simulink model "god"  (R2018a)
settings: Solver=VariableStepAuto  StartTime=0.0  StopTime=10  FixedStep=0.01  RelTol=1e-3
libraries: instrumentlib x15
settings Model: EnablePacing=on  Creator=U500304  LastModifiedBy=U500304
settings SolverCC: ZeroCrossAlgorithm=Adaptive
settings DataIOCC: SaveOutput=off  SaveTime=off
settings DebuggingCC: MaxConsecutiveZCsMsg=none

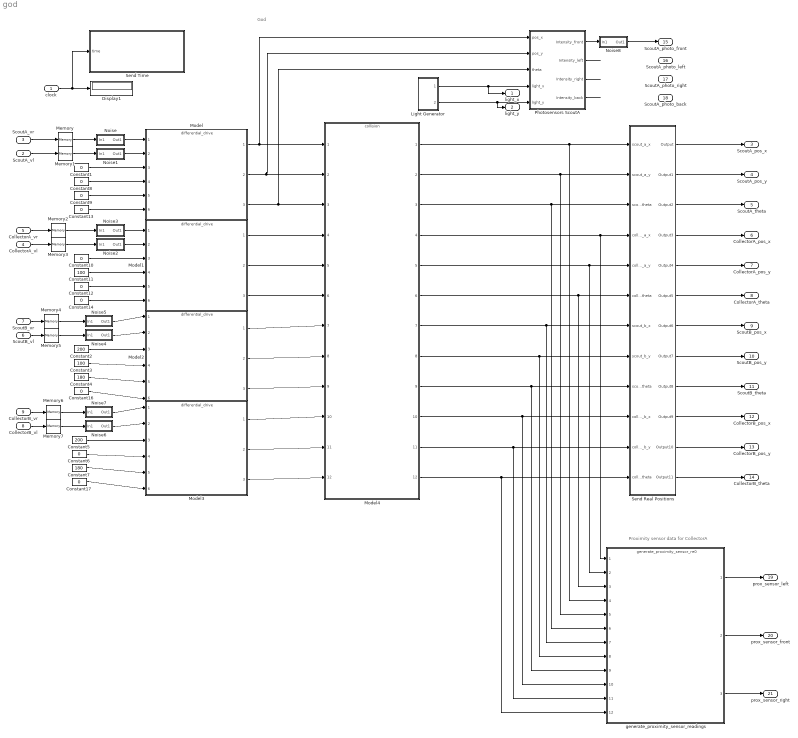
== system god ==
  note: Proximity sensor data for CollectorA
  note: God
  clock : Inport  OutDataTypeStr=double  PortDimensions=1  SampleTime=0
  ScoutA_vl : Inport  Port=2
  ScoutA_vr : Inport  Port=3
  CollectorA_vl : Inport  Port=4
  CollectorA_vr : Inport  Port=5
  ScoutB_vl : Inport  Port=6
  ScoutB_vr : Inport  Port=7
  CollectorB_vl : Inport  Port=8
  CollectorB_vr : Inport  Port=9
  Constant{1,6,8..10,12..14,16..17} (10 alike) : Constant  Value=0
  Constant11 : Constant  Value=100
  Constant2 : Constant  Value=200
  Constant3 : Constant  Value=100
  Constant4 : Constant  Value=180
  Constant5 : Constant  Value=200
  Constant7 : Constant  Value=180
  Display1 : Display
  Light Generator : Subsystem
  Memory{,1..7} (8 alike) : Memory
  Model{,1..3} (4 alike) : ModelReference  ModelNameDialog=differential_drive.slx  SimulationMode=Normal  ModelReferenceVersion=1.313
  Model4 : ModelReference  ModelNameDialog=collision.slx  SimulationMode=Normal  ModelReferenceVersion=1.672
  Noise : Subsystem
  Noise1 : Subsystem
  Noise2 : Subsystem
  Noise3 : Subsystem
  Noise4 : Subsystem
  Noise5 : Subsystem
  Noise6 : Subsystem
  Noise7 : Subsystem
  Noise8 : Subsystem
  Photosensors ScoutA : Subsystem
  Send Real Positions : Subsystem
  Send Time : Subsystem
  generate_proximity_sensor_readings : ModelReference  ModelNameDialog=generate_proximity_sensor_re0  SimulationMode=Normal  ModelReferenceVersion=1.659
  light_x : Outport
  light_y : Outport  Port=2
  ScoutA_pos_x : Outport  Port=3
  ScoutA_pos_y : Outport  Port=4
  ScoutA_theta : Outport  Port=5
  CollectorA_pos_x : Outport  Port=6
  CollectorA_pos_y : Outport  Port=7
  CollectorA_theta : Outport  Port=8
  ScoutB_pos_x : Outport  Port=9
  ScoutB_pos_y : Outport  Port=10
  ScoutB_theta : Outport  Port=11
  CollectorB_pos_x : Outport  Port=12
  CollectorB_pos_y : Outport  Port=13
  CollectorB_theta : Outport  Port=14
  ScoutA_photo_front : Outport  Port=15
  ScoutA_photo_left : Outport  Port=16
  ScoutA_photo_right : Outport  Port=17
  ScoutA_photo_back : Outport  Port=18
  prox_sensor_left : Outport  Port=19
  prox_sensor_front : Outport  Port=20
  prox_sensor_right : Outport  Port=21
  wires:
  clock/1 -> Send Time/1(time), Display1/1
  Constant9/1 -> Model/5
  Constant1/1 -> Model/3
  Constant8/1 -> Model/4
  Constant11/1 -> Model1/4
  Constant10/1 -> Model1/3
  Constant12/1 -> Model1/5
  ScoutB_vl/1 -> Memory5/1
  ScoutB_vr/1 -> Memory4/1
  Constant4/1 -> Model2/5
  Constant2/1 -> Model2/3
  Constant3/1 -> Model2/4
  Constant6/1 -> Model3/4
  Constant7/1 -> Model3/5
  Constant5/1 -> Model3/3
  CollectorB_vl/1 -> Memory7/1
  CollectorB_vr/1 -> Memory6/1
  Noise5/1(Out1) -> Model2/1
  Noise4/1(Out1) -> Model2/2
  Noise6/1(Out1) -> Model3/2
  Noise7/1(Out1) -> Model3/1
  Light Generator/1(Light_x) -> light_x/1, Photosensors ScoutA/4(light_x)
  Light Generator/2(Light_y) -> light_y/1, Photosensors ScoutA/5(light_y)
  Photosensors ScoutA/1(Intensity_front) -> Noise8/1(In1)
  Photosensors ScoutA/2(Intensity_left) -> ?
  Photosensors ScoutA/3(Intensity_right) -> ?
  Photosensors ScoutA/4(Intensity_back) -> ?
  Noise/1(Out1) -> Model/1
  Noise1/1(Out1) -> Model/2
  Noise2/1(Out1) -> Model1/2
  Noise3/1(Out1) -> Model1/1
  Model/3 -> Photosensors ScoutA/3(theta), Model4/3
  Model/2 -> Photosensors ScoutA/2(pos_y), Model4/2
  Model/1 -> Photosensors ScoutA/1(pos_x), Model4/1
  ScoutA_vr/1 -> Memory/1
  ScoutA_vl/1 -> Memory1/1
  CollectorA_vr/1 -> Memory2/1
  CollectorA_vl/1 -> Memory3/1
  Memory/1 -> Noise/1(In1)
  Memory1/1 -> Noise1/1(In1)
  Memory2/1 -> Noise3/1(In1)
  Memory3/1 -> Noise2/1(In1)
  Constant13/1 -> Model/6
  Constant14/1 -> Model1/6
  Constant16/1 -> Model2/6
  Constant17/1 -> Model3/6
  Model4/11 -> generate_proximity_sensor_readings/11, Send Real Positions/11(collector_b_y)
  Model4/10 -> generate_proximity_sensor_readings/10, Send Real Positions/10(collector_b_x)
  Model4/9 -> generate_proximity_sensor_readings/9, Send Real Positions/9(scout_b_theta)
  Model4/8 -> generate_proximity_sensor_readings/8, Send Real Positions/8(scout_b_y)
  Model4/7 -> generate_proximity_sensor_readings/7, Send Real Positions/7(scout_b_x)
  Model4/12 -> generate_proximity_sensor_readings/12, Send Real Positions/12(collector_b_theta)
  Memory5/1 -> Noise4/1(In1)
  Memory4/1 -> Noise5/1(In1)
  Memory6/1 -> Noise7/1(In1)
  Memory7/1 -> Noise6/1(In1)
  Model1/1 -> Model4/4
  Model1/2 -> Model4/5
  Model1/3 -> Model4/6
  Model2/1 -> Model4/7
  Model2/2 -> Model4/8
  Model2/3 -> Model4/9
  Model3/1 -> Model4/10
  Model3/2 -> Model4/11
  Model3/3 -> Model4/12
  Send Real Positions/1(Output) -> ScoutA_pos_x/1
  Send Real Positions/2(Output1) -> ScoutA_pos_y/1
  Send Real Positions/3(Output2) -> ScoutA_theta/1
  Send Real Positions/4(Output3) -> CollectorA_pos_x/1
  Send Real Positions/5(Output4) -> CollectorA_pos_y/1
  Send Real Positions/6(Output5) -> CollectorA_theta/1
  Send Real Positions/7(Output6) -> ScoutB_pos_x/1
  Send Real Positions/8(Output7) -> ScoutB_pos_y/1
  Send Real Positions/9(Output8) -> ScoutB_theta/1
  Send Real Positions/10(Output9) -> CollectorB_pos_x/1
  Send Real Positions/11(Output10) -> CollectorB_pos_y/1
  Send Real Positions/12(Output11) -> CollectorB_theta/1
  Model4/2 -> generate_proximity_sensor_readings/5, Send Real Positions/2(scout_a_y)
  Model4/3 -> generate_proximity_sensor_readings/6, Send Real Positions/3(scout_a_theta)
  Model4/4 -> generate_proximity_sensor_readings/1, Send Real Positions/4(collector_a_x)
  Model4/5 -> generate_proximity_sensor_readings/2, Send Real Positions/5(collector_a_y)
  Model4/6 -> generate_proximity_sensor_readings/3, Send Real Positions/6(collector_a_theta)
  generate_proximity_sensor_readings/1 -> prox_sensor_left/1
  generate_proximity_sensor_readings/2 -> prox_sensor_front/1
  generate_proximity_sensor_readings/3 -> prox_sensor_right/1
  Model4/1 -> generate_proximity_sensor_readings/4, Send Real Positions/1(scout_a_x)
  Noise8/1(Out1) -> ScoutA_photo_front/1
  ? -> ScoutA_photo_left/1
  ? -> ScoutA_photo_right/1
  ? -> ScoutA_photo_back/1

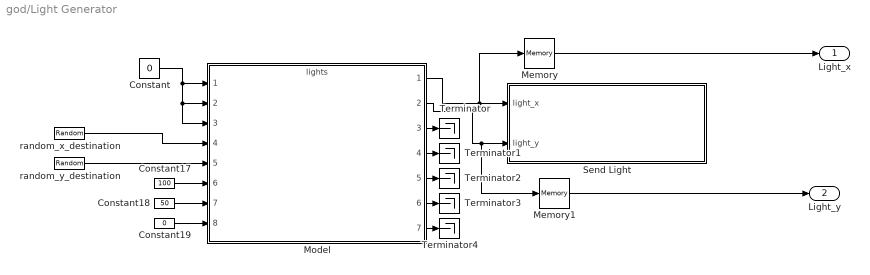
== system god/Light Generator ==
  Constant : Constant  Value=0
  Constant17 : Constant  Value=100
  Constant18 : Constant  Value=50
  Constant19 : Constant  Value=0
  Memory : Memory
  Memory1 : Memory
  Model : ModelReference  ModelNameDialog=lights  SimulationMode=Normal  ModelReferenceVersion=1.293
  Send Light : Subsystem
  Terminator{,1..4} (5 alike) : Terminator
  random_x_destination : UniformRandomNumber  Minimum=0  Maximum=199  Seed=14  SampleTime=1
  random_y_destination : UniformRandomNumber  Minimum=0  Maximum=99  Seed=66  SampleTime=1
  Light_x : Outport
  Light_y : Outport  Port=2
  wires:
  Model/3 -> Terminator/1
  Constant17/1 -> Model/6
  random_y_destination/1 -> Model/5
  Model/6 -> Terminator3/1
  Constant19/1 -> Model/8
  Memory1/1 -> Light_y/1
  Constant/1 -> Model/1, Model/3, Model/2
  Model/4 -> Terminator1/1
  Model/1 -> Memory/1, Send Light/1(light_x)
  Model/2 -> Memory1/1, Send Light/2(light_y)
  random_x_destination/1 -> Model/4
  Model/5 -> Terminator2/1
  Model/7 -> Terminator4/1
  Constant18/1 -> Model/7
  Memory/1 -> Light_x/1

== system god/Noise ==
  In1 : Inport
  Add : Sum
  Multiply : Product
  Uniform Random Number : UniformRandomNumber  Minimum=-0.02  Maximum=0.02  SampleTime=0.1
  Out1 : Outport
  wires:
  Multiply/1 -> Add/1
  In1/1 -> Add/2, Multiply/2
  Uniform Random Number/1 -> Multiply/1
  Add/1 -> Out1/1

== system god/Noise1 ==
  In1 : Inport
  Add : Sum
  Multiply : Product
  Uniform Random Number : UniformRandomNumber  Minimum=-0.02  Maximum=0.02  Seed=1  SampleTime=0.1
  Out1 : Outport
  wires:
  Add/1 -> Out1/1
  Uniform Random Number/1 -> Multiply/1
  In1/1 -> Multiply/2, Add/2
  Multiply/1 -> Add/1

== system god/Noise2 ==
  In1 : Inport
  Add : Sum
  Multiply : Product
  Uniform Random Number : UniformRandomNumber  Minimum=-0.02  Maximum=0.02  SampleTime=0.1
  Out1 : Outport
  wires:
  Add/1 -> Out1/1
  Uniform Random Number/1 -> Multiply/1
  In1/1 -> Multiply/2, Add/2
  Multiply/1 -> Add/1

== system god/Noise3 ==
  In1 : Inport
  Add : Sum
  Multiply : Product
  Uniform Random Number : UniformRandomNumber  Minimum=-0.02  Maximum=0.02  SampleTime=0.1
  Out1 : Outport
  wires:
  Multiply/1 -> Add/1
  In1/1 -> Add/2, Multiply/2
  Uniform Random Number/1 -> Multiply/1
  Add/1 -> Out1/1

== system god/Noise4 ==
  In1 : Inport
  Add : Sum
  Multiply : Product
  Uniform Random Number : UniformRandomNumber  Minimum=-0.02  Maximum=0.02  Seed=2  SampleTime=0.1
  Out1 : Outport
  wires:
  Multiply/1 -> Add/1
  In1/1 -> Add/2, Multiply/2
  Uniform Random Number/1 -> Multiply/1
  Add/1 -> Out1/1

== system god/Noise5 ==
  In1 : Inport
  Add : Sum
  Multiply : Product
  Uniform Random Number : UniformRandomNumber  Minimum=-0.02  Maximum=0.02  Seed=3  SampleTime=0.1
  Out1 : Outport
  wires:
  Add/1 -> Out1/1
  Uniform Random Number/1 -> Multiply/1
  In1/1 -> Multiply/2, Add/2
  Multiply/1 -> Add/1

== system god/Noise6 ==
  In1 : Inport
  Add : Sum
  Multiply : Product
  Uniform Random Number : UniformRandomNumber  Minimum=-0.02  Maximum=0.02  Seed=4  SampleTime=0.1
  Out1 : Outport
  wires:
  Add/1 -> Out1/1
  Uniform Random Number/1 -> Multiply/1
  In1/1 -> Multiply/2, Add/2
  Multiply/1 -> Add/1

== system god/Noise7 ==
  In1 : Inport
  Add : Sum
  Multiply : Product
  Uniform Random Number : UniformRandomNumber  Minimum=-0.02  Maximum=0.02  Seed=5  SampleTime=0.1
  Out1 : Outport
  wires:
  Multiply/1 -> Add/1
  In1/1 -> Add/2, Multiply/2
  Uniform Random Number/1 -> Multiply/1
  Add/1 -> Out1/1

== system god/Noise8 ==
  In1 : Inport
  Add : Sum
  Constant : Constant  Value=255
  Constant1 : Constant  Value=0
  Multiply : Product
  Switch : Switch  Criteria=u2 > Threshold  Threshold=255
  Switch1 : Switch  Criteria=u2 > Threshold
  Uniform Random Number : UniformRandomNumber  Minimum=-0.04  Maximum=0.04  SampleTime=0.1
  Out1 : Outport
  wires:
  Uniform Random Number/1 -> Multiply/1
  In1/1 -> Multiply/2, Add/2
  Multiply/1 -> Add/1
  Add/1 -> Switch/3
  Constant/1 -> Switch/1, Switch/2
  Switch/1 -> Switch1/1
  Constant1/1 -> Switch1/2, Switch1/3
  Switch1/1 -> Out1/1

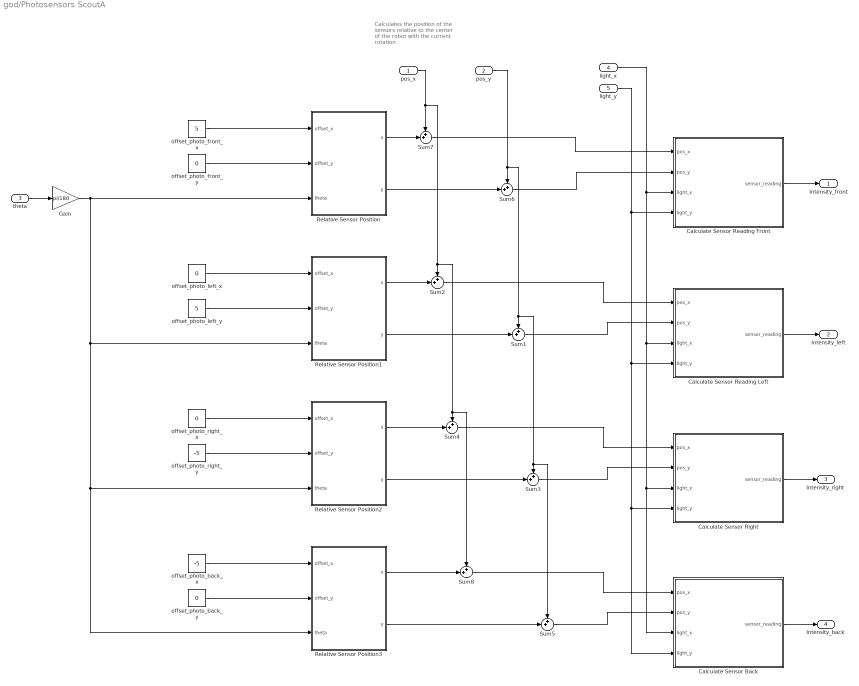
== system god/Photosensors ScoutA ==
  note: Calculates the position of
      | the sensors relative to the
      | center of the robot with the
      | current rotation
  pos_x : Inport
  pos_y : Inport  Port=2
  theta : Inport  Port=3
  light_x : Inport  Port=4
  light_y : Inport  Port=5
  Calculate Sensor Back : Subsystem
  Calculate Sensor Reading Front : Subsystem
  Calculate Sensor Reading Left : Subsystem
  Calculate Sensor Right : Subsystem
  Gain : Gain  Gain=pi/180
  Relative Sensor Position : Subsystem  TreatAsAtomicUnit=on
  Relative Sensor Position1 : Subsystem
  Relative Sensor Position2 : Subsystem
  Relative Sensor Position3 : Subsystem
  Sum{1..8} (8 alike) : Sum  Inputs=++|
  offset_photo_back_x : Constant  Value=-5
  offset_photo_back_y : Constant  Value=0
  offset_photo_front_x : Constant  Value=5
  offset_photo_front_y : Constant  Value=0
  offset_photo_left_x : Constant  Value=0
  offset_photo_left_y : Constant  Value=5
  offset_photo_right_x : Constant  Value=0
  offset_photo_right_y : Constant  Value=-5
  Intensity_front : Outport
  Intensity_left : Outport  Port=2
  Intensity_right : Outport  Port=3
  Intensity_back : Outport  Port=4
  wires:
  offset_photo_front_x/1 -> Relative Sensor Position/1(offset_x)
  offset_photo_front_y/1 -> Relative Sensor Position/2(offset_y)
  Relative Sensor Position/2(y) -> Sum6/2
  Calculate Sensor Reading Front/1(sensor_reading) -> Intensity_front/1
  Sum6/1 -> Calculate Sensor Reading Front/2(pos_y)
  Sum7/1 -> Calculate Sensor Reading Front/1(pos_x)
  offset_photo_left_y/1 -> Relative Sensor Position1/2(offset_y)
  offset_photo_left_x/1 -> Relative Sensor Position1/1(offset_x)
  Relative Sensor Position/1(x) -> Sum7/2
  Relative Sensor Position1/1(x) -> Sum2/2
  Relative Sensor Position1/2(y) -> Sum1/2
  Sum1/1 -> Calculate Sensor Reading Left/2(pos_y)
  Sum2/1 -> Calculate Sensor Reading Left/1(pos_x)
  offset_photo_right_y/1 -> Relative Sensor Position2/2(offset_y)
  offset_photo_right_x/1 -> Relative Sensor Position2/1(offset_x)
  Relative Sensor Position2/1(x) -> Sum4/2
  Sum4/1 -> Calculate Sensor Right/1(pos_x)
  Sum3/1 -> Calculate Sensor Right/2(pos_y)
  Relative Sensor Position2/2(y) -> Sum3/2
  light_y/1 -> Calculate Sensor Back/4(light_y), Calculate Sensor Right/4(light_y), Calculate Sensor Reading Left/4(light_y), Calculate Sensor Reading Front/4(light_y)
  Relative Sensor Position3/2(y) -> Sum5/2
  pos_y/1 -> Sum6/1, Sum5/1, Sum3/1, Sum1/1
  Sum5/1 -> Calculate Sensor Back/2(pos_y)
  Sum8/1 -> Calculate Sensor Back/1(pos_x)
  Gain/1 -> Relative Sensor Position3/3(theta), Relative Sensor Position2/3(theta), Relative Sensor Position1/3(theta), Relative Sensor Position/3(theta)
  Relative Sensor Position3/1(x) -> Sum8/2
  offset_photo_back_x/1 -> Relative Sensor Position3/1(offset_x)
  offset_photo_back_y/1 -> Relative Sensor Position3/2(offset_y)
  light_x/1 -> Calculate Sensor Back/3(light_x), Calculate Sensor Right/3(light_x), Calculate Sensor Reading Left/3(light_x), Calculate Sensor Reading Front/3(light_x)
  pos_x/1 -> Sum8/1, Sum4/1, Sum2/1, Sum7/1
  Calculate Sensor Reading Left/1(sensor_reading) -> Intensity_left/1
  Calculate Sensor Right/1(sensor_reading) -> Intensity_right/1
  Calculate Sensor Back/1(sensor_reading) -> Intensity_back/1
  theta/1 -> Gain/1

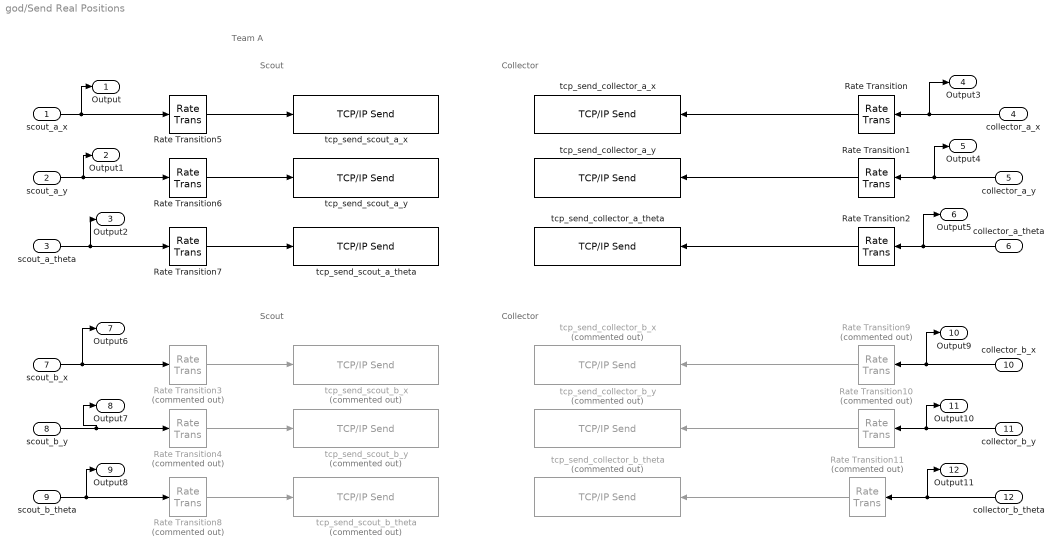
== system god/Send Real Positions ==
  note: Team A
  note: Scout
  note: Collector
  note: Scout
  note: Collector
  scout_a_x : Inport
  scout_a_y : Inport  Port=2
  scout_a_theta : Inport  Port=3
  collector_a_x : Inport  Port=4
  collector_a_y : Inport  Port=5
  collector_a_theta : Inport  Port=6
  scout_b_x : Inport  Port=7
  scout_b_y : Inport  Port=8
  scout_b_theta : Inport  Port=9
  collector_b_x : Inport  Port=10
  collector_b_y : Inport  Port=11
  collector_b_theta : Inport  Port=12
  Rate Transition{,1..2,5..7} (6 alike) : RateTransition  OutPortSampleTime=0.05
  Rate Transition{3..4,8..11} (6 alike) : RateTransition  Commented=on  OutPortSampleTime=0.1
  tcp_send_collector_a_theta : instrumentlib/TCP//IP Send  Host=localhost  Port=50034  EnableBlockingMode=off  Timeout=1  ByteOrder=LittleEndian  TransferDelay=on
      settings: SourceProductName=Instrument Control Toolbox
  tcp_send_collector_a_x : instrumentlib/TCP//IP Send  Host=localhost  Port=50032  EnableBlockingMode=off  Timeout=1  ByteOrder=LittleEndian  TransferDelay=on
      settings: SourceProductName=Instrument Control Toolbox
  tcp_send_collector_a_y : instrumentlib/TCP//IP Send  Host=localhost  Port=50033  EnableBlockingMode=off  Timeout=1  ByteOrder=LittleEndian  TransferDelay=on
      settings: SourceProductName=Instrument Control Toolbox
  tcp_send_collector_b_theta : instrumentlib/TCP//IP Send  Commented=on  Host=localhost  Port=50012  EnableBlockingMode=on  Timeout=1  ByteOrder=LittleEndian  TransferDelay=on
      settings: SourceProductName=Instrument Control Toolbox
  tcp_send_collector_b_x : instrumentlib/TCP//IP Send  Commented=on  Host=localhost  Port=50010  EnableBlockingMode=on  Timeout=1  ByteOrder=LittleEndian  TransferDelay=on
      settings: SourceProductName=Instrument Control Toolbox
  tcp_send_collector_b_y : instrumentlib/TCP//IP Send  Commented=on  Host=localhost  Port=50011  EnableBlockingMode=on  Timeout=1  ByteOrder=LittleEndian  TransferDelay=on
      settings: SourceProductName=Instrument Control Toolbox
  tcp_send_scout_a_theta : instrumentlib/TCP//IP Send  Host=localhost  Port=50031  EnableBlockingMode=off  Timeout=1  ByteOrder=LittleEndian  TransferDelay=on
      settings: SourceProductName=Instrument Control Toolbox
  tcp_send_scout_a_x : instrumentlib/TCP//IP Send  Host=localhost  Port=50029  EnableBlockingMode=off  Timeout=1  ByteOrder=LittleEndian  TransferDelay=on
      settings: SourceProductName=Instrument Control Toolbox
  tcp_send_scout_a_y : instrumentlib/TCP//IP Send  Host=localhost  Port=50030  EnableBlockingMode=off  Timeout=1  ByteOrder=LittleEndian  TransferDelay=on
      settings: SourceProductName=Instrument Control Toolbox
  tcp_send_scout_b_theta : instrumentlib/TCP//IP Send  Commented=on  Host=localhost  Port=50009  EnableBlockingMode=on  Timeout=1  ByteOrder=LittleEndian  TransferDelay=on
      settings: SourceProductName=Instrument Control Toolbox
  tcp_send_scout_b_x : instrumentlib/TCP//IP Send  Commented=on  Host=localhost  Port=50007  EnableBlockingMode=on  Timeout=1  ByteOrder=LittleEndian  TransferDelay=on
      settings: SourceProductName=Instrument Control Toolbox
  tcp_send_scout_b_y : instrumentlib/TCP//IP Send  Commented=on  Host=localhost  Port=50008  EnableBlockingMode=on  Timeout=1  ByteOrder=LittleEndian  TransferDelay=on
      settings: SourceProductName=Instrument Control Toolbox
  Output : Outport
  Output1 : Outport  Port=2
  Output2 : Outport  Port=3
  Output3 : Outport  Port=4
  Output4 : Outport  Port=5
  Output5 : Outport  Port=6
  Output6 : Outport  Port=7
  Output7 : Outport  Port=8
  Output8 : Outport  Port=9
  Output9 : Outport  Port=10
  Output10 : Outport  Port=11
  Output11 : Outport  Port=12
  wires:
  collector_b_x/1 -> Output9/1, Rate Transition9/1
  scout_a_x/1 -> Output/1, Rate Transition5/1
  collector_b_y/1 -> Output10/1, Rate Transition10/1
  scout_a_y/1 -> Output1/1, Rate Transition6/1
  collector_a_y/1 -> Output4/1, Rate Transition1/1
  collector_a_theta/1 -> Output5/1, Rate Transition2/1
  collector_b_theta/1 -> Output11/1, Rate Transition11/1
  scout_a_theta/1 -> Output2/1, Rate Transition7/1
  scout_b_theta/1 -> Output8/1, Rate Transition8/1
  scout_b_y/1 -> Output7/1, Rate Transition4/1
  scout_b_x/1 -> Output6/1, Rate Transition3/1
  Rate Transition/1 -> tcp_send_collector_a_x/1
  Rate Transition1/1 -> tcp_send_collector_a_y/1
  Rate Transition2/1 -> tcp_send_collector_a_theta/1
  Rate Transition5/1 -> tcp_send_scout_a_x/1
  Rate Transition6/1 -> tcp_send_scout_a_y/1
  Rate Transition7/1 -> tcp_send_scout_a_theta/1
  Rate Transition3/1 -> tcp_send_scout_b_x/1
  Rate Transition4/1 -> tcp_send_scout_b_y/1
  Rate Transition8/1 -> tcp_send_scout_b_theta/1
  Rate Transition9/1 -> tcp_send_collector_b_x/1
  Rate Transition10/1 -> tcp_send_collector_b_y/1
  Rate Transition11/1 -> tcp_send_collector_b_theta/1
  collector_a_x/1 -> Output3/1, Rate Transition/1

== system god/Send Time ==
  note: Light
  time : Inport
  Rate Transition8 : RateTransition  OutPortSampleTime=0.1
  tcp_send_light_x : instrumentlib/TCP//IP Send  Host=localhost  Port=50021  EnableBlockingMode=on  Timeout=1  ByteOrder=LittleEndian  TransferDelay=on
      settings: SourceProductName=Instrument Control Toolbox
  wires:
  Rate Transition8/1 -> tcp_send_light_x/1
  time/1 -> Rate Transition8/1

== system god/Light Generator/Send Light ==
  note: Light
  light_x : Inport
  light_y : Inport  Port=2
  Rate Transition8 : RateTransition  OutPortSampleTime=0.1
  Rate Transition9 : RateTransition  OutPortSampleTime=0.1
  tcp_send_light_x : instrumentlib/TCP//IP Send  Host=localhost  Port=50013  EnableBlockingMode=off  Timeout=1  ByteOrder=LittleEndian  TransferDelay=on
      settings: SourceProductName=Instrument Control Toolbox
  tcp_send_light_y : instrumentlib/TCP//IP Send  Host=localhost  Port=50014  EnableBlockingMode=off  Timeout=1  ByteOrder=LittleEndian  TransferDelay=on
      settings: SourceProductName=Instrument Control Toolbox
  wires:
  light_y/1 -> Rate Transition9/1
  light_x/1 -> Rate Transition8/1
  Rate Transition8/1 -> tcp_send_light_x/1
  Rate Transition9/1 -> tcp_send_light_y/1

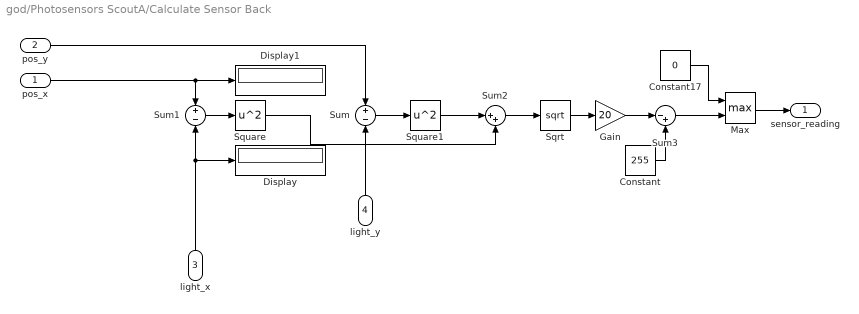
== system god/Photosensors ScoutA/Calculate Sensor Back ==
  pos_x : Inport
  pos_y : Inport  Port=2
  light_x : Inport  Port=3
  light_y : Inport  Port=4
  Constant : Constant  Value=255
  Constant17 : Constant  Value=0
  Display : Display
  Display1 : Display
  Gain : Gain  Gain=20
  Max : MinMax  Function=max  Inputs=2
  Sqrt : Sqrt  SaturateOnIntegerOverflow=on
  Square : Math  Operator=square  SaturateOnIntegerOverflow=on
  Square1 : Math  Operator=square  SaturateOnIntegerOverflow=on
  Sum : Sum  Inputs=+-
  Sum1 : Sum  Inputs=+-
  Sum2 : Sum  Inputs=|++
  Sum3 : Sum  Inputs=|-+
  sensor_reading : Outport
  wires:
  Constant17/1 -> Max/1
  pos_x/1 -> Display1/1, Sum1/1
  light_x/1 -> Display/1, Sum1/2
  Gain/1 -> Sum3/1
  light_y/1 -> Sum/2
  Constant/1 -> Sum3/2
  Square/1 -> Sum2/2
  Sum2/1 -> Sqrt/1
  Max/1 -> sensor_reading/1
  Square1/1 -> Sum2/1
  Sum/1 -> Square1/1
  Sum3/1 -> Max/2
  Sum1/1 -> Square/1
  Sqrt/1 -> Gain/1
  pos_y/1 -> Sum/1

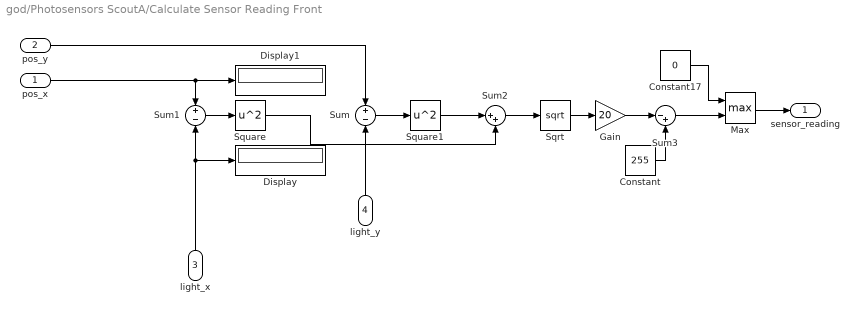
== system god/Photosensors ScoutA/Calculate Sensor Reading Front ==
  pos_x : Inport
  pos_y : Inport  Port=2
  light_x : Inport  Port=3
  light_y : Inport  Port=4
  Constant : Constant  Value=255
  Constant17 : Constant  Value=0
  Display : Display
  Display1 : Display
  Gain : Gain  Gain=20
  Max : MinMax  Function=max  Inputs=2
  Sqrt : Sqrt  SaturateOnIntegerOverflow=on
  Square : Math  Operator=square  SaturateOnIntegerOverflow=on
  Square1 : Math  Operator=square  SaturateOnIntegerOverflow=on
  Sum : Sum  Inputs=+-
  Sum1 : Sum  Inputs=+-
  Sum2 : Sum  Inputs=|++
  Sum3 : Sum  Inputs=|-+
  sensor_reading : Outport
  wires:
  Constant17/1 -> Max/1
  pos_x/1 -> Display1/1, Sum1/1
  light_x/1 -> Display/1, Sum1/2
  Gain/1 -> Sum3/1
  light_y/1 -> Sum/2
  Constant/1 -> Sum3/2
  Square/1 -> Sum2/2
  Sum2/1 -> Sqrt/1
  Max/1 -> sensor_reading/1
  Square1/1 -> Sum2/1
  Sum/1 -> Square1/1
  Sum3/1 -> Max/2
  Sum1/1 -> Square/1
  Sqrt/1 -> Gain/1
  pos_y/1 -> Sum/1

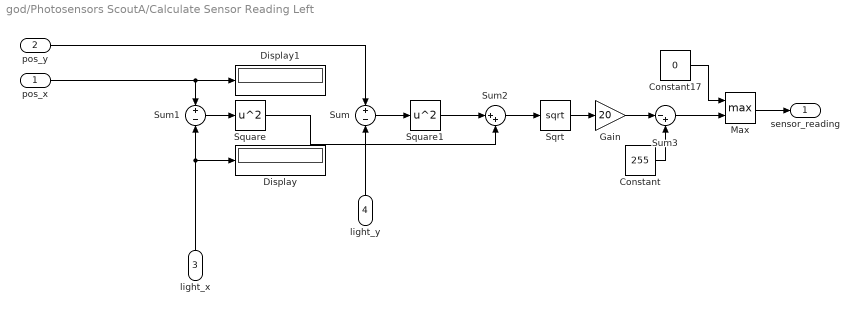
== system god/Photosensors ScoutA/Calculate Sensor Reading Left ==
  pos_x : Inport
  pos_y : Inport  Port=2
  light_x : Inport  Port=3
  light_y : Inport  Port=4
  Constant : Constant  Value=255
  Constant17 : Constant  Value=0
  Display : Display
  Display1 : Display
  Gain : Gain  Gain=20
  Max : MinMax  Function=max  Inputs=2
  Sqrt : Sqrt  SaturateOnIntegerOverflow=on
  Square : Math  Operator=square  SaturateOnIntegerOverflow=on
  Square1 : Math  Operator=square  SaturateOnIntegerOverflow=on
  Sum : Sum  Inputs=+-
  Sum1 : Sum  Inputs=+-
  Sum2 : Sum  Inputs=|++
  Sum3 : Sum  Inputs=|-+
  sensor_reading : Outport
  wires:
  pos_y/1 -> Sum/1
  Sqrt/1 -> Gain/1
  Sum1/1 -> Square/1
  Sum3/1 -> Max/2
  Sum/1 -> Square1/1
  Square1/1 -> Sum2/1
  Max/1 -> sensor_reading/1
  Sum2/1 -> Sqrt/1
  Square/1 -> Sum2/2
  Constant/1 -> Sum3/2
  light_y/1 -> Sum/2
  Gain/1 -> Sum3/1
  light_x/1 -> Sum1/2, Display/1
  pos_x/1 -> Sum1/1, Display1/1
  Constant17/1 -> Max/1

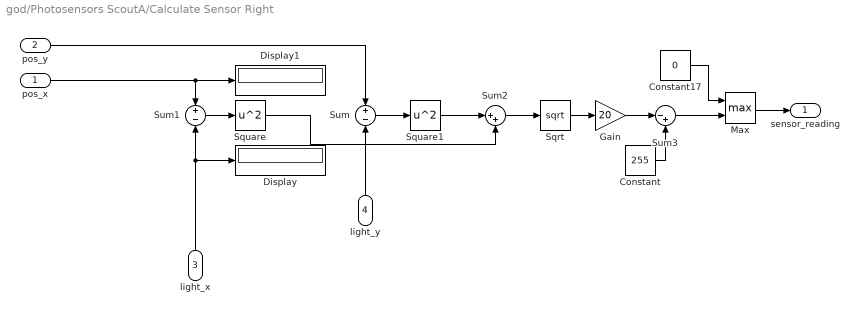
== system god/Photosensors ScoutA/Calculate Sensor Right ==
  pos_x : Inport
  pos_y : Inport  Port=2
  light_x : Inport  Port=3
  light_y : Inport  Port=4
  Constant : Constant  Value=255
  Constant17 : Constant  Value=0
  Display : Display
  Display1 : Display
  Gain : Gain  Gain=20
  Max : MinMax  Function=max  Inputs=2
  Sqrt : Sqrt  SaturateOnIntegerOverflow=on
  Square : Math  Operator=square  SaturateOnIntegerOverflow=on
  Square1 : Math  Operator=square  SaturateOnIntegerOverflow=on
  Sum : Sum  Inputs=+-
  Sum1 : Sum  Inputs=+-
  Sum2 : Sum  Inputs=|++
  Sum3 : Sum  Inputs=|-+
  sensor_reading : Outport
  wires:
  pos_y/1 -> Sum/1
  Sqrt/1 -> Gain/1
  Sum1/1 -> Square/1
  Sum3/1 -> Max/2
  Sum/1 -> Square1/1
  Square1/1 -> Sum2/1
  Max/1 -> sensor_reading/1
  Sum2/1 -> Sqrt/1
  Square/1 -> Sum2/2
  Constant/1 -> Sum3/2
  light_y/1 -> Sum/2
  Gain/1 -> Sum3/1
  light_x/1 -> Sum1/2, Display/1
  pos_x/1 -> Sum1/1, Display1/1
  Constant17/1 -> Max/1

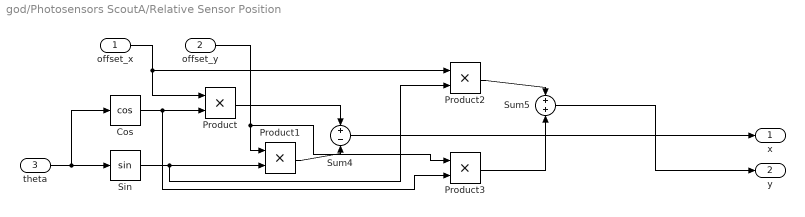
== system god/Photosensors ScoutA/Relative Sensor Position ==
  offset_x : Inport
  offset_y : Inport  Port=2
  theta : Inport  Port=3
  Cos : Trigonometry  Operator=cos
  Product{,1..3} (4 alike) : Product
  Sin : Trigonometry
  Sum4 : Sum  Inputs=+-
  Sum5 : Sum
  x : Outport
  y : Outport  Port=2
  wires:
  Sin/1 -> Product2/2, Product1/2
  Cos/1 -> Product/2, Product3/2
  Product/1 -> Sum4/1
  offset_y/1 -> Product3/1, Product1/1
  offset_x/1 -> Product/1, Product2/1
  theta/1 -> Cos/1, Sin/1
  Product2/1 -> Sum5/1
  Product1/1 -> Sum4/2
  Product3/1 -> Sum5/2
  Sum5/1 -> y/1
  Sum4/1 -> x/1

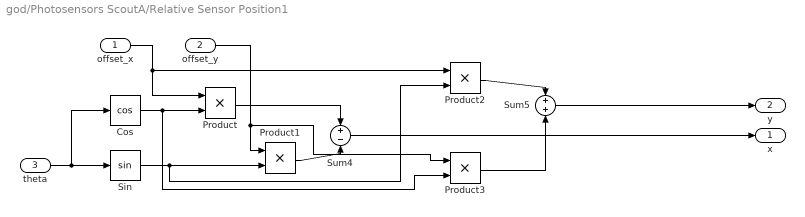
== system god/Photosensors ScoutA/Relative Sensor Position1 ==
  offset_x : Inport
  offset_y : Inport  Port=2
  theta : Inport  Port=3
  Cos : Trigonometry  Operator=cos
  Product{,1..3} (4 alike) : Product
  Sin : Trigonometry
  Sum4 : Sum  Inputs=+-
  Sum5 : Sum
  x : Outport
  y : Outport  Port=2
  wires:
  Sum4/1 -> x/1
  Sum5/1 -> y/1
  Product3/1 -> Sum5/2
  Product1/1 -> Sum4/2
  Product2/1 -> Sum5/1
  theta/1 -> Sin/1, Cos/1
  offset_x/1 -> Product2/1, Product/1
  offset_y/1 -> Product1/1, Product3/1
  Product/1 -> Sum4/1
  Cos/1 -> Product3/2, Product/2
  Sin/1 -> Product1/2, Product2/2

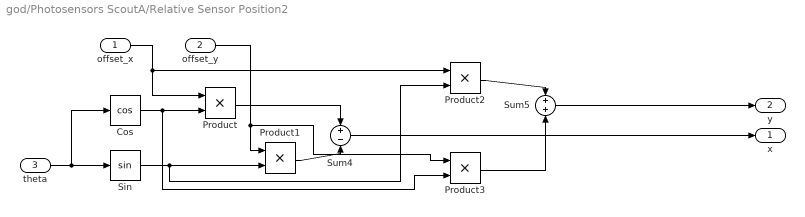
== system god/Photosensors ScoutA/Relative Sensor Position2 ==
  offset_x : Inport
  offset_y : Inport  Port=2
  theta : Inport  Port=3
  Cos : Trigonometry  Operator=cos
  Product{,1..3} (4 alike) : Product
  Sin : Trigonometry
  Sum4 : Sum  Inputs=+-
  Sum5 : Sum
  x : Outport
  y : Outport  Port=2
  wires:
  Sum4/1 -> x/1
  Sum5/1 -> y/1
  Product3/1 -> Sum5/2
  Product1/1 -> Sum4/2
  Product2/1 -> Sum5/1
  theta/1 -> Sin/1, Cos/1
  offset_x/1 -> Product2/1, Product/1
  offset_y/1 -> Product1/1, Product3/1
  Product/1 -> Sum4/1
  Cos/1 -> Product3/2, Product/2
  Sin/1 -> Product1/2, Product2/2

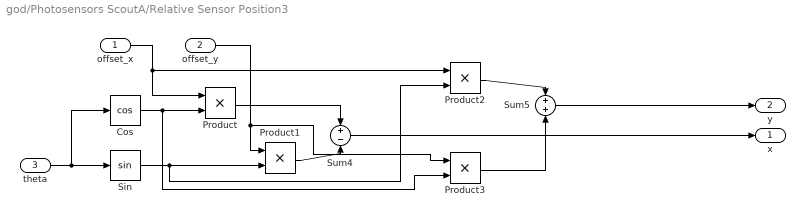
== system god/Photosensors ScoutA/Relative Sensor Position3 ==
  offset_x : Inport
  offset_y : Inport  Port=2
  theta : Inport  Port=3
  Cos : Trigonometry  Operator=cos
  Product{,1..3} (4 alike) : Product
  Sin : Trigonometry
  Sum4 : Sum  Inputs=+-
  Sum5 : Sum
  x : Outport
  y : Outport  Port=2
  wires:
  Sin/1 -> Product2/2, Product1/2
  Cos/1 -> Product/2, Product3/2
  Product/1 -> Sum4/1
  offset_y/1 -> Product3/1, Product1/1
  offset_x/1 -> Product/1, Product2/1
  theta/1 -> Cos/1, Sin/1
  Product2/1 -> Sum5/1
  Product1/1 -> Sum4/2
  Product3/1 -> Sum5/2
  Sum5/1 -> y/1
  Sum4/1 -> x/1
